simulink model "chair"  (R2024b)
settings: Solver=ode4  StartTime=0.0  StopTime=60  FixedStep=1e-4  RelTol=1e-3
values from neighbouring files (symbols this model uses):
  g = 9,81    [params.m]
  G_r = 32    [params.m]
  Ke_motor = 0.05    [params.m]
  Kt_motor = 0.05    [params.m]
  L = 0.50    (= 0.5)    [params.m]
  l1 = 0.30    (= 0.3)    [params.m]
  l2 = 0.20    (= 0.2)    [params.m]
  L_motor = 0.0003    [params.m]
  m = 180    [params.m]
  mu = 0.015    [params.m]
  r = 0.25    [params.m]
  R_motor = 0.15    [params.m]
  V_max = 24    [params.m]
  v_s = 0.05    [params.m]
libraries: slpidlib x1, simulink x1
settings Model: Creator=pedro-cruz  LastModifiedBy=pedro-cruz

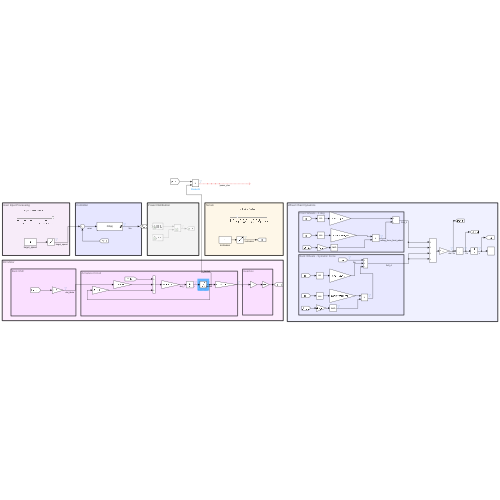
[thumbnail: Simulink's stored preview of the top-level diagram]
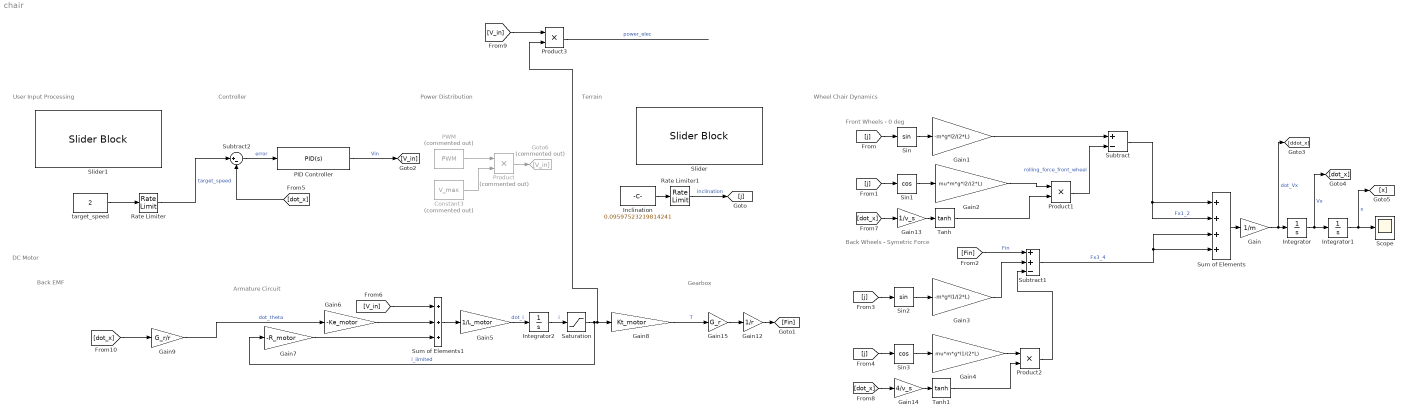
== system chair ==
  note: User Input Processing
  note: Controller
  note: Power Distribution
  note: DC Motor
  note: Back EMF
  note: Terrain
  note: Wheel Chair Dynamics
  note: Back Wheels - Symetric Force
  note: Front Wheels - 0 deg
  note: Armature Circuit
  note: Gearbox
  Constant3 : Constant  Commented=on  Value=V_max
  Gain : Gain  Gain=1/m
  Gain1 : Gain  Gain=-m*g*l2/(2*L)
  Gain12 : Gain  Gain=1/r
  Gain13 : Gain  Gain=1/v_s
  Gain14 : Gain  Gain=4/v_s
  Gain15 : Gain  Gain=G_r
  Gain2 : Gain  Gain=mu*m*g*l2/(2*L)
  Gain3 : Gain  Gain=-m*g*l1/(2*L)
  Gain4 : Gain  Gain=mu*m*g*l1/(2*L)
  Gain5 : Gain  Gain=1/L_motor
  Gain6 : Gain  Gain=-Ke_motor
  Gain7 : Gain  Gain=-R_motor
  Gain8 : Gain  Gain=Kt_motor
  Gain9 : Gain  Gain=G_r/r
  Goto6 : Goto  Commented=on  GotoTag=V_in
  Inclination : Constant  Value=0.09597523219814241
  Integrator : Integrator
  Integrator1 : Integrator
  Integrator2 : Integrator
  PID Controller : slpidlib/PID Controller  Controller=PID  Form=Ideal  TimeDomain=Continuous-time  UseExternalTs=off  SampleTime=-1  IntegratorMethod=Forward Euler  FilterMethod=Forward Euler  ControllerParametersSource=internal  P=53  I=18.9  UseKiTs=off  D=0  UseExternalDerivativeSource=off  N=100  UseFilter=on  TunerSelectOption=Transfer Function Based (PID Tuner App)  InitialConditionSource=internal  InitialConditionForIntegrator=0  InitialConditionForFilter=0  DifferentiatorICPrevScaledInput=0  ExternalReset=none  TrackingMode=off  Kt=1  LimitOutput=on  SatLimitsSource=internal  UpperSaturationLimit=V_max  LowerSaturationLimit=-V_max  LinearizeAsGain=on  AntiWindupMode=clamping  Kb=1  LimitIntegrator=off  UpperIntegratorSaturationLimit=inf  LowerIntegratorSaturationLimit=-inf  POutMin=[]  POutMax=[]  IOutMin=[]  IOutMax=[]  DOutMin=[]  DOutMax=[]  NOutMin=[]  NOutMax=[]  SumOutMin=[]  SumOutMax=[]  SaturationOutMin=[]  SaturationOutMax=[]  PParamMin=[]  PParamMax=[]  IParamMin=[]  IParamMax=[]  DParamMin=[]  DParamMax=[]  NParamMin=[]  NParamMax=[]  KbParamMin=[]  KbParamMax=[]  KtParamMin=[]  KtParamMax=[]  KbOutMin=[]  KbOutMax=[]  KtOutMin=[]  KtOutMax=[]  IntegratorOutMin=[]  IntegratorOutMax=[]  FilterOutMin=[]  FilterOutMax=[]  SumI1OutMin=[]  SumI1OutMax=[]  SumI2OutMin=[]  SumI2OutMax=[]  SumI3OutMin=[]  SumI3OutMax=[]  SumI4OutMin=[]  SumI4OutMax=[]  SumDOutMin=[]  SumDOutMax=[]  DifferentiatorOutMin=[]  DifferentiatorOutMax=[]  FilterDiffOutCoefMin=[]  FilterDiffOutCoefMax=[]  ReciprocalOutMin=[]  ReciprocalOutMax=[]  SumDenOutMin=[]  SumDenOutMax=[]  SumNumOutMin=[]  SumNumOutMax=[]  DivideOutMin=[]  DivideOutMax=[]  UdiffTsProdOutMin=[]  UdiffTsProdOutMax=[]  NTsProdOutMin=[]  NTsProdOutMax=[]  UintegralTsProdOutMin=[]  UintegralTsProdOutMax=[]  UngainTsProdOutMin=[]  UngainTsProdOutMax=[]  ClampingZeroOutDataTypeStr=Inherit: Inherit via back propagation  ClampingZeroOutMin=[]  ClampingZeroOutMax=[]  FilterDenConstantOutDataTypeStr=Inherit: Inherit via back propagation  FilterDenConstantOutMin=[]  FilterDenConstantOutMax=[]  PCopyOutDataTypeStr=Inherit: Inherit via back propagation  PCopyOutMin=[]  PCopyOutMax=[]  NCopyOutDataTypeStr=Inherit: Inherit via back propagation  NCopyOutMin=[]  NCopyOutMax=[]  IntegratorContinuousStateAttributes=''  IntegratorStateMustResolveToSignalObject=off  IntegratorRTWStateStorageClass=Auto  FilterContinuousStateAttributes=''  FilterStateMustResolveToSignalObject=off  FilterRTWStateStorageClass=Auto  ParallelPVariant=Passthrough  IdealPVariant=InternalParameters  IVariant=InternalParameters  DVariant=InternalParameters  IntegratorVariant=Continuous  SatVariant=Enabled  AWVariant=ContClampingIdeal  PCopyVariant=InternalParamsIdeal  TRVariant=Disabled  FdbkBlocksVariant=Forward  IdealPFdbkVariant=Disabled  SatFdbkVariant=Disabled  DerivativeFilterVariant=ContFilter  NVariant=InternalParameters  NCopyVariant=Disabled  FilterICVariant=InternalICsFilter  IntegratorICVariant=InternalICs  ExternalResetVariant=Disabled  TRSumVariant=Passthrough  SumFdbkVariant=Disabled  SumVariant=Sum_PID  TsampFilterVariant=InternalTs  TsampNgainVariant=Passthrough  TsampIntegralVariant=Disabled_SignalSpec  ExternalSaturationOutDataTypeStr=Inherit: Same as second input  DerivativeSourceVariant=ErrorSignal  PreIntVariant=InternalPreInt
  PWM : simulink/Discontinuities/PWM  Commented=on  DisableCoverage=on  Period=0.1  InitialDelay=0  DisallowZeroDutyCycle=off  RunAtFixedTimeIntervals=on  SampleTime=0.001
  Product : Product  Commented=on
  Product1 : Product
  Product2 : Product
  Product3 : Product
  Rate Limiter : RateLimiter  RisingSlewLimit=0.1  SampleTimeMode=inherited
  Rate Limiter1 : RateLimiter  RisingSlewLimit=0.3  SampleTimeMode=inherited
  Saturation : Saturate  UpperLimit=30  LowerLimit=-20
  Scope : Scope
  Sin : Trigonometry
  Sin1 : Trigonometry  Operator=cos
  Sin2 : Trigonometry
  Sin3 : Trigonometry  Operator=cos
  Slider : SliderBlock  ScaleMax=0.5
  Slider1 : SliderBlock  ScaleMax=2
  Subtract : Sum  Inputs=+-
  Subtract1 : Sum  Inputs=++-
  Subtract2 : Sum  Inputs=|+-
  Sum of Elements : Sum  Inputs=++++
  Sum of Elements1 : Sum  Inputs=+++
  Tanh : Trigonometry  Operator=tanh
  Tanh1 : Trigonometry  Operator=tanh
  target_speed : Constant  Value=2
  wires:
  Integrator/1 -> [dot_x], Integrator1/1  "Vx"
  Gain/1 -> [ddot_x], Integrator/1  "dot_Vx"
  Sum of Elements/1 -> Gain/1
  [j] -> Sin/1
  Gain1/1 -> Subtract/1
  Sin/1 -> Gain1/1
  [j] -> Sin1/1
  Sin1/1 -> Gain2/1
  Subtract/1 -> Sum of Elements/2, Sum of Elements/1  "Fx1_2"
  [Fin] -> Subtract1/1  "Fin"
  [j] -> Sin2/1
  Sin2/1 -> Gain3/1
  [j] -> Sin3/1
  Sin3/1 -> Gain4/1
  Subtract1/1 -> Sum of Elements/4, Sum of Elements/3  "Fx3_4"
  Integrator1/1 -> Scope/1, [x]  "x"
  Inclination/1 -> Rate Limiter1/1
  Integrator2/1 -> Saturation/1  "i"
  Gain5/1 -> Integrator2/1  "dot_i"
  Sum of Elements1/1 -> Gain5/1
  [V_in] -> Sum of Elements1/1
  Gain6/1 -> Sum of Elements1/2
  Gain7/1 -> Sum of Elements1/3
  Gain8/1 -> Gain15/1  "T"
  Subtract2/1 -> PID Controller/1  "error"
  [dot_x] -> Subtract2/2
  PWM/1 -> Product/1
  Constant3/1 -> Product/2
  Product/1 -> Goto6/1
  target_speed/1 -> Rate Limiter/1
  Gain12/1 -> [Fin]
  PID Controller/1 -> [V_in]  "Vin"
  Rate Limiter/1 -> Subtract2/1  "target_speed"
  Gain2/1 -> Product1/1
  [dot_x] -> Gain13/1
  Gain13/1 -> Tanh/1
  Gain4/1 -> Product2/1
  [dot_x] -> Gain14/1
  Gain14/1 -> Tanh1/1
  Tanh1/1 -> Product2/2
  Gain15/1 -> Gain12/1
  [V_in] -> Product3/1
  Product3/1 -> ?  "power_elec"
  Rate Limiter1/1 -> [j]  "inclination"
  Gain3/1 -> Subtract1/2
  Product2/1 -> Subtract1/3
  Product1/1 -> Subtract/2  "rolling_force_front_wheel"
  Tanh/1 -> Product1/2
  [dot_x] -> Gain9/1
  Gain9/1 -> Gain6/1  "dot_theta"
  Saturation/1 -> Gain7/1, Gain8/1, Product3/2  "i_limited"
